simulink model "cca_nmpc_closed_loop"  (R2025a)
settings: Solver=FixedStepDiscrete  StartTime=0.0  StopTime=2  FixedStep=0.1  RelTol=1e-3
settings Model: Creator=thientn204  LastModifiedBy=thientn204

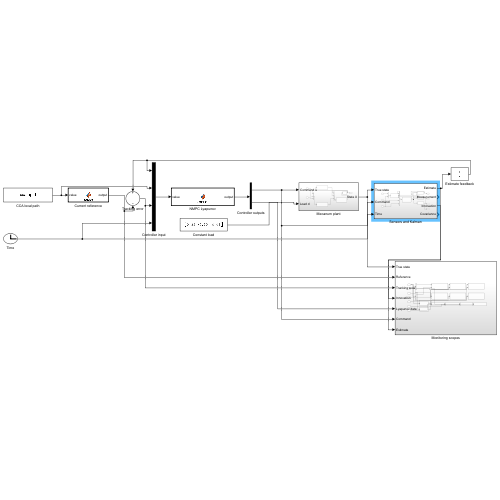
[thumbnail: Simulink's stored preview of the top-level diagram]
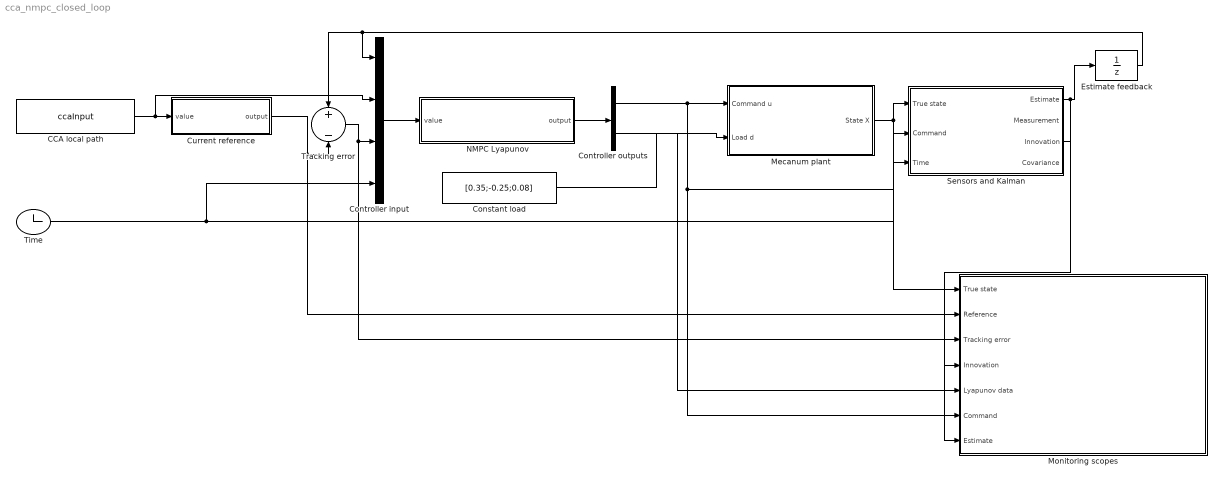
== system cca_nmpc_closed_loop ==
  CCA local path : FromWorkspace  VariableName=ccaInput  OutputAfterFinalValue=Holding final value
  Constant load : Constant  Value=[0.35;-0.25;0.08]
  Controller input : Mux
  Controller outputs : Demux  Outputs=[3 9]
  Current reference : MATLAB Function  TreatAsAtomicUnit=on
  Estimate feedback : UnitDelay  InitialCondition=[0;0;0;0;0;0]  SampleTime=0.1  HasFrameUpgradeWarning=on
  Mecanum plant : Subsystem
  Monitoring scopes : Subsystem
  NMPC Lyapunov : MATLAB Function  TreatAsAtomicUnit=on
  Sensors and Kalman : Subsystem
  Time : Clock
  Tracking error : Sum  Inputs=+-
  wires:
  CCA local path/1 -> Current reference/1(value), Controller input/2
  Current reference/1(output) -> Tracking error/2, Monitoring scopes/2(Reference)
  Sensors and Kalman/1(Estimate) -> Estimate feedback/1, Monitoring scopes/7(Estimate)
  Estimate feedback/1 -> Tracking error/1, Controller input/1
  Tracking error/1 -> Controller input/3, Monitoring scopes/3(Tracking error)
  Time/1 -> Controller input/4, Sensors and Kalman/3(Time)
  Controller input/1 -> NMPC Lyapunov/1(value)
  NMPC Lyapunov/1(output) -> Controller outputs/1
  Controller outputs/1 -> Sensors and Kalman/2(Command), Monitoring scopes/6(Command), Mecanum plant/1(Command u)
  Constant load/1 -> Mecanum plant/2(Load d)
  Mecanum plant/1(State X) -> Sensors and Kalman/1(True state), Monitoring scopes/1(True state)
  Sensors and Kalman/3(Innovation) -> Monitoring scopes/4(Innovation)
  Controller outputs/2 -> Monitoring scopes/5(Lyapunov data)

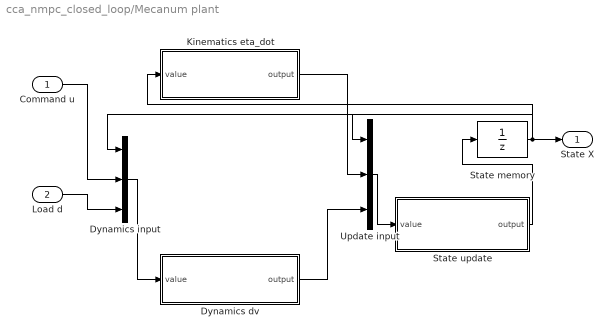
== system cca_nmpc_closed_loop/Mecanum plant ==
  Command u : Inport
  Load d : Inport  Port=2
  Dynamics dv : MATLAB Function  TreatAsAtomicUnit=on
  Dynamics input : Mux  Inputs=3
  Kinematics eta_dot : MATLAB Function  TreatAsAtomicUnit=on
  State memory : UnitDelay  InitialCondition=[0;0;0;0;0;0]  SampleTime=0.1  HasFrameUpgradeWarning=on
  State update : MATLAB Function  TreatAsAtomicUnit=on
  Update input : Mux  Inputs=3
  State X : Outport
  wires:
  Command u/1 -> Dynamics input/2
  Load d/1 -> Dynamics input/3
  State memory/1 -> Kinematics eta_dot/1(value), Dynamics input/1, Update input/1, State X/1
  Dynamics input/1 -> Dynamics dv/1(value)
  Kinematics eta_dot/1(output) -> Update input/2
  Dynamics dv/1(output) -> Update input/3
  Update input/1 -> State update/1(value)
  State update/1(output) -> State memory/1

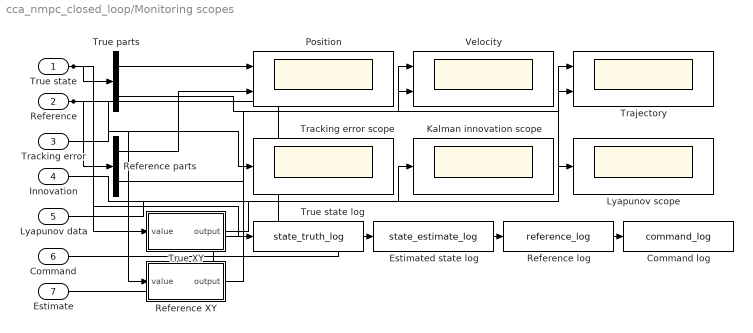
== system cca_nmpc_closed_loop/Monitoring scopes ==
  True state : Inport
  Reference : Inport  Port=2
  Tracking error : Inport  Port=3
  Innovation : Inport  Port=4
  Lyapunov data : Inport  Port=5
  Command : Inport  Port=6
  Estimate : Inport  Port=7
  Command log : ToWorkspace  VariableName=command_log  SaveFormat=Timeseries  SampleTime=-1
  Estimated state log : ToWorkspace  VariableName=state_estimate_log  SaveFormat=Timeseries  SampleTime=-1
  Kalman innovation scope : Scope
  Lyapunov scope : Scope
  Position : Scope  NumInputPorts=2
  Reference XY : MATLAB Function  TreatAsAtomicUnit=on
  Reference log : ToWorkspace  VariableName=reference_log  SaveFormat=Timeseries  SampleTime=-1
  Reference parts : Demux  Outputs=[3 3]
  Tracking error scope : Scope
  Trajectory : Scope  NumInputPorts=2
  True XY : MATLAB Function  TreatAsAtomicUnit=on
  True parts : Demux  Outputs=[3 3]
  True state log : ToWorkspace  VariableName=state_truth_log  SaveFormat=Timeseries  SampleTime=-1
  Velocity : Scope  NumInputPorts=2
  wires:
  True state/1 -> True parts/1, True XY/1(value), True state log/1
  Reference/1 -> Reference parts/1, Reference XY/1(value), Reference log/1
  True parts/1 -> Position/1
  Reference parts/1 -> Position/2
  True parts/2 -> Velocity/1
  Reference parts/2 -> Velocity/2
  True XY/1(output) -> Trajectory/1
  Reference XY/1(output) -> Trajectory/2
  Tracking error/1 -> Tracking error scope/1
  Innovation/1 -> Kalman innovation scope/1
  Lyapunov data/1 -> Lyapunov scope/1
  Command/1 -> Command log/1
  Estimate/1 -> Estimated state log/1

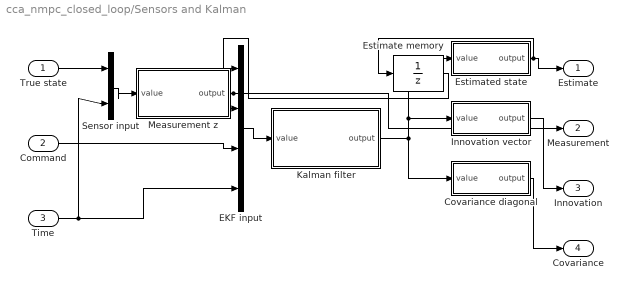
== system cca_nmpc_closed_loop/Sensors and Kalman ==
  True state : Inport
  Command : Inport  Port=2
  Time : Inport  Port=3
  Covariance diagonal : MATLAB Function  TreatAsAtomicUnit=on
  EKF input : Mux
  Estimate memory : UnitDelay  InitialCondition=[0;0;0;0;0;0]  SampleTime=0.1  HasFrameUpgradeWarning=on
  Estimated state : MATLAB Function  TreatAsAtomicUnit=on
  Innovation vector : MATLAB Function  TreatAsAtomicUnit=on
  Kalman filter : MATLAB Function  TreatAsAtomicUnit=on
  Measurement z : MATLAB Function  TreatAsAtomicUnit=on
  Sensor input : Mux  Inputs=2
  Estimate : Outport
  Measurement : Outport  Port=2
  Innovation : Outport  Port=3
  Covariance : Outport  Port=4
  wires:
  True state/1 -> Sensor input/1
  Time/1 -> Sensor input/2, EKF input/4
  Sensor input/1 -> Measurement z/1(value)
  Measurement z/1(output) -> EKF input/2, Measurement/1
  Estimate memory/1 -> EKF input/1
  Command/1 -> EKF input/3
  EKF input/1 -> Kalman filter/1(value)
  Kalman filter/1(output) -> Estimated state/1(value), Innovation vector/1(value), Covariance diagonal/1(value)
  Estimated state/1(output) -> Estimate memory/1, Estimate/1
  Innovation vector/1(output) -> Innovation/1
  Covariance diagonal/1(output) -> Covariance/1

== matlab function cca_nmpc_closed_loop/Current reference ==
  data: value input; output output
function output = select(value)
output = value(1:6);
end

== matlab function cca_nmpc_closed_loop/Mecanum plant/Kinematics eta_dot ==
  data: value input; output output
function output = kinematics_block(value)
coder.extrinsic('kinematics');
output = zeros(3,1);
state = value(1:6);
output = kinematics(state, state(4:6), 'world');
end

== matlab function cca_nmpc_closed_loop/Mecanum plant/Dynamics dv ==
  data: value input; output output
function output = dynamics_block(value)
coder.extrinsic('dynamics','robot_parameters');
output = zeros(3,1);
p = robot_parameters();
output = dynamics(value(1:6), value(7:9), value(10:12), p);
end

== matlab function cca_nmpc_closed_loop/Mecanum plant/State update ==
  data: value input; output output
function output = update(value)
coder.extrinsic('wrap_angle');
output = value(1:6) + 0.1 * [value(7:9); value(10:12)];
output(3) = wrap_angle(output(3));
end

== matlab function cca_nmpc_closed_loop/Sensors and Kalman/Measurement z ==
  data: value input; output output
function output = measure(value)
coder.extrinsic('sensor_model','robot_parameters');
output = zeros(6,1);
output = sensor_model(value(1:6), value(7), robot_parameters());
end

== matlab function cca_nmpc_closed_loop/Sensors and Kalman/Kalman filter ==
  data: value input; output output
function output = filter(value)
coder.extrinsic('simulation.simulinkEkfStep');
output = zeros(19,1);
output = simulation.simulinkEkfStep(value);
end

== matlab function cca_nmpc_closed_loop/Sensors and Kalman/Estimated state ==
  data: value input; output output
function output = state(value)
output = value(1:6);
end

== matlab function cca_nmpc_closed_loop/Sensors and Kalman/Innovation vector ==
  data: value input; output output
function output = innovation(value)
output = value(7:12);
end

== matlab function cca_nmpc_closed_loop/NMPC Lyapunov ==
  data: value input; output output
function output = control(value)
coder.extrinsic('simulation.simulinkNmpcStep');
output = zeros(12,1);
output = simulation.simulinkNmpcStep(value);
end

== matlab function cca_nmpc_closed_loop/Sensors and Kalman/Covariance diagonal ==
  data: value input; output output
function output = covariance(value)
output = value(13:18);
end

== matlab function cca_nmpc_closed_loop/Monitoring scopes/True XY ==
  data: value input; output output
function output = xy(value)
output = value(1:2);
end

== matlab function cca_nmpc_closed_loop/Monitoring scopes/Reference XY ==
  data: value input; output output
function output = xy(value)
output = value(1:2);
end
